simulink model "sistemaLinearOrdem3"  (R2018b)
settings: Solver=ode45  StartTime=0.0  StopTime=10.0  RelTol=1e-3
values from neighbouring files (symbols this model uses):
  p = linspace(0.1,1.2,50)    [atividade1.m]
settings Model: Creator=joaol  LastModifiedBy=bryan

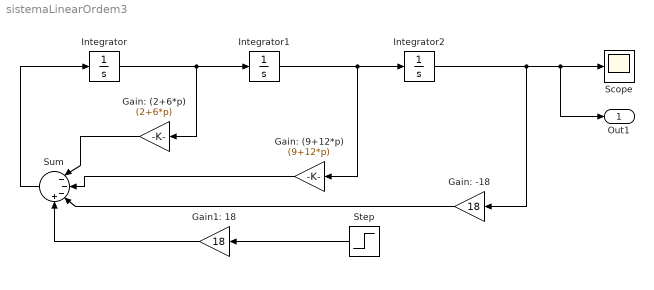
== system sistemaLinearOrdem3 ==
  Gain1: 18 : Gain  Gain=18
  Gain: (2+6*p) : Gain  Gain=(2+6*p)
  "Gain: (9+12*p) " : Gain  Gain=(9+12*p)
  Gain: -18 : Gain  Gain=18
  Integrator : Integrator
  Integrator1 : Integrator
  Integrator2 : Integrator
  Scope : Scope
  Step : Step  Time=0.01  SampleTime=0
  Sum : Sum  Inputs=|---+
  Out1 : Outport  SignalName=y(t)
  wires:
  Integrator/1 -> Gain: (2+6*p)/1, Integrator1/1
  Integrator1/1 -> "Gain: (9+12*p) "/1, Integrator2/1
  Integrator2/1 -> Gain: -18/1, Out1/1, Scope/1
  Sum/1 -> Integrator/1
  Gain: (2+6*p)/1 -> Sum/1
  "Gain: (9+12*p) "/1 -> Sum/2
  Gain: -18/1 -> Sum/3
  Step/1 -> Gain1: 18/1
  Gain1: 18/1 -> Sum/4
